simulink model "testwintrack2"  (R2021b)
settings: Solver=ode45  StartTime=0.0  StopTime=100  MaxStep=0.01  RelTol=1e-3
libraries: aerolibconvert2 x4, simulink x1
settings Model: Creator=cigla  LastModifiedBy=eforce

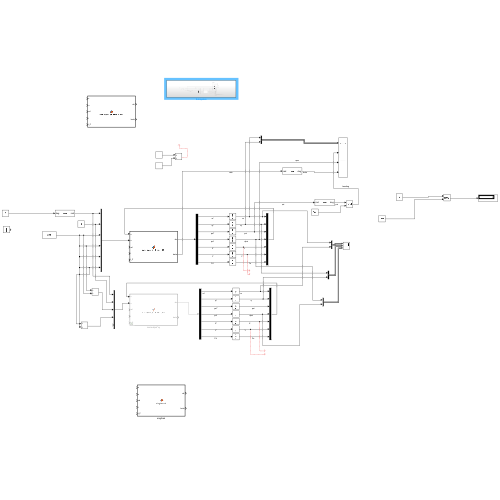
[thumbnail: Simulink's stored preview of the top-level diagram]
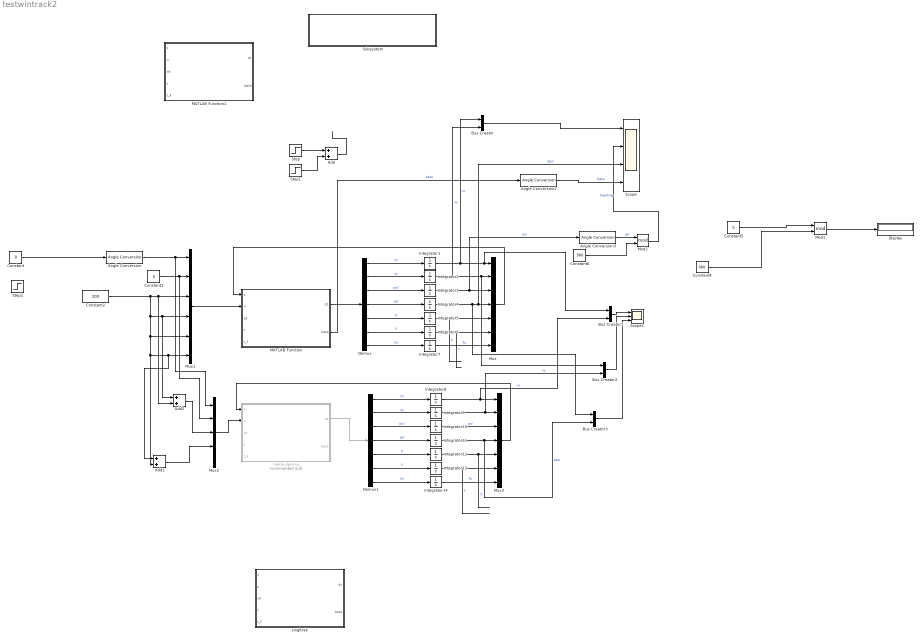
== system testwintrack2 ==
  Add : Sum
  Add1 : Sum
  Add2 : Sum
  Angle Conversion : aerolibconvert2/Angle Conversion  IU=deg  OU=rad
  Angle Conversion2 : aerolibconvert2/Angle Conversion  IU=rad  OU=deg
  Angle Conversion3 : aerolibconvert2/Angle Conversion  IU=rad  OU=deg
  Bus Creator{,1..3} (4 alike) : BusCreator  Inputs=2
  Constant : Constant  Value=0
  Constant1 : Constant  Value=0
  Constant2 : Constant  Value=200
  Constant4 : Constant  Value=360
  Constant5 : Constant  Value=5
  Constant6 : Constant  Value=360
  Demux : Demux  Outputs=7
  Demux1 : Demux  Outputs=7
  Display : Display
  Integrator{1..14} (14 alike) : Integrator
  MATLAB Function : MATLAB Function  TreatAsAtomicUnit=on
  MATLAB Function1 : MATLAB Function  TreatAsAtomicUnit=on
  Mod1 : Math  Operator=mod  SaturateOnIntegerOverflow=on
  Mod2 : Math  Operator=mod  SaturateOnIntegerOverflow=on
  Mux : Mux  Inputs=7
  Mux1 : Mux  Inputs=6
  Mux2 : Mux  Inputs=5
  Mux3 : Mux  Inputs=7
  Scope : Scope  NumInputPorts=4
  Scope1 : Scope  NumInputPorts=3
  Step : Step  Time=10  After=15  SampleTime=0
  Step1 : Step  Time=11  After=-30  SampleTime=0
  Step2 : Step  Time=10  After=20  SampleTime=0
  Subsystem : Subsystem
  nema dpsi*vy : MATLAB Function  Commented=on  TreatAsAtomicUnit=on
  singltrak : MATLAB Function  TreatAsAtomicUnit=on
  wires:
  MATLAB Function/1(dz) -> Demux/1
  Mux/1 -> MATLAB Function/1(z)
  Mux1/1 -> MATLAB Function/2(u)
  Demux/1 -> Integrator1/1  "vx'"
  Demux/2 -> Integrator2/1  "vy'"
  Demux/3 -> Integrator3/1  "psi''"
  Demux/4 -> Integrator4/1  "psi'"
  Demux/5 -> Integrator5/1  "X'"
  Demux/6 -> Integrator6/1  "Y'"
  Demux/7 -> Integrator7/1  "Fz'"
  Integrator1/1 -> Bus Creator/1, Bus Creator1/1, Mux/1  "vx"
  Integrator2/1 -> Bus Creator/2, Bus Creator2/1, Mux/2  "vy"
  Integrator7/1 -> Mux/7  "Fz"
  Integrator6/1 -> Mux/6  "Y"
  Integrator5/1 -> Mux/5  "X"
  Integrator4/1 -> Bus Creator3/1, Scope/3, Mux/4  "dpsi"
  Integrator3/1 -> Angle Conversion3/1, Mux/3  "psi"
  Add/1 -> ?
  Constant1/1 -> Mux2/2, Mux1/2
  Constant2/1 -> Add1/2, Add1/1, Mux1/6, Mux1/5, Add2/1, Mux1/4, Add2/2, Mux1/3
  Angle Conversion/1 -> Mux2/1, Mux1/1
  Step/1 -> Add/1
  Step1/1 -> Add/2
  Constant/1 -> Angle Conversion/1
  Bus Creator/1 -> Scope/1
  MATLAB Function/2(beta) -> Angle Conversion2/1  "beta"
  Angle Conversion2/1 -> Scope/4  "beta"
  Constant4/1 -> Mod1/2
  Constant5/1 -> Mod1/1
  Mod1/1 -> Display/1
  Angle Conversion3/1 -> Mod2/1  "psi"
  Constant6/1 -> Mod2/2
  Mod2/1 -> Scope/2  "heading"
  Add2/1 -> Mux2/3
  Add1/1 -> Mux2/4
  Mux2/1 -> nema dpsi*vy/2(u)
  Demux1/2 -> Integrator9/1  "vy'"
  Integrator14/1 -> Mux3/7  "Fz"
  Integrator12/1 -> Mux3/5  "X"
  Integrator10/1 -> Mux3/3  "psi"
  Integrator13/1 -> Mux3/6  "Y"
  Integrator9/1 -> Bus Creator2/2, Mux3/2  "vy"
  Demux1/5 -> Integrator12/1  "X'"
  Mux3/1 -> nema dpsi*vy/1(z)
  Demux1/7 -> Integrator14/1  "Fz'"
  Demux1/4 -> Integrator11/1  "psi'"
  Demux1/3 -> Integrator10/1  "psi''"
  Integrator11/1 -> Bus Creator3/2, Mux3/4  "dpsi"
  nema dpsi*vy/1(dz) -> Demux1/1
  Demux1/6 -> Integrator13/1  "Y'"
  Demux1/1 -> Integrator8/1  "vx'"
  Integrator8/1 -> Bus Creator1/2, Mux3/1  "vx"
  Bus Creator1/1 -> Scope1/1
  Bus Creator2/1 -> Scope1/2
  Bus Creator3/1 -> Scope1/3

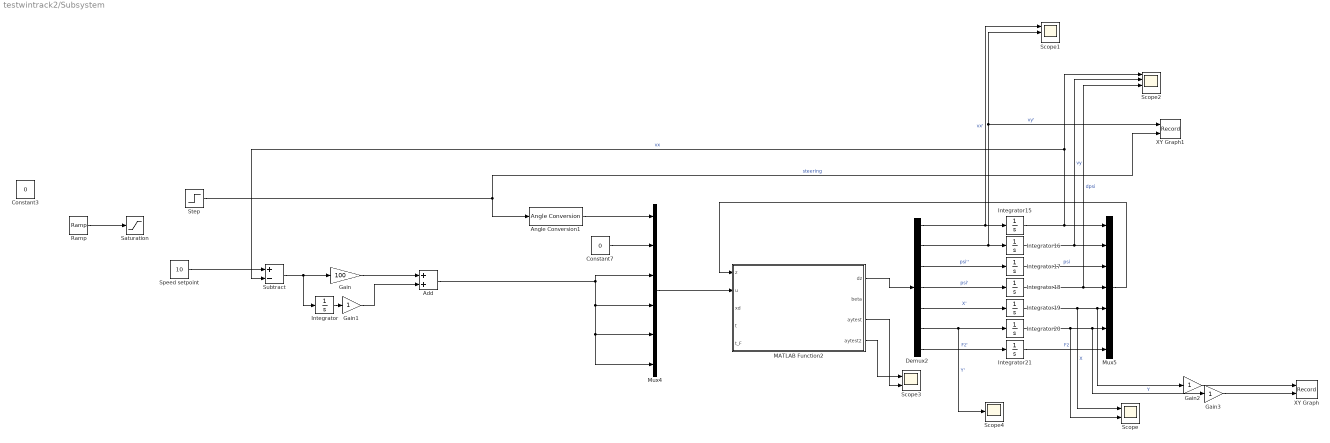
== system testwintrack2/Subsystem ==
  Add : Sum
  Angle Conversion1 : aerolibconvert2/Angle Conversion  IU=deg  OU=rad
  Constant3 : Constant  Value=0
  Constant7 : Constant  Value=0
  Demux2 : Demux  Outputs=7
  Gain : Gain  Gain=100
  Gain1 : Gain
  Gain2 : Gain
  Gain3 : Gain
  Integrator : Integrator  UpperSaturationLimit=10  LowerSaturationLimit=-10
  Integrator{15..21} (7 alike) : Integrator
  MATLAB Function2 : MATLAB Function  TreatAsAtomicUnit=on
  Mux4 : Mux  Inputs=6
  Mux5 : Mux  Inputs=7
  Ramp : simulink/Sources/Ramp  slope=1  start=30  InitialOutput=0
  Saturation : Saturate  UpperLimit=20  LowerLimit=-20
  Scope : Scope  NumInputPorts=2
  Scope1 : Scope  NumInputPorts=3
  Scope2 : Scope  NumInputPorts=4
  Scope3 : Scope  NumInputPorts=2
  Scope4 : Scope
  Speed setpoint : Constant  Value=10
  Step : Step  Time=10  After=10  SampleTime=0
  Subtract : Sum  Inputs=+-
  XY Graph : Record  FileSettingsInternal="{\"entries\":[{\"content\":{\"excelSettings\":{\"content\":{},\"type\":\"Streamout.ExcelSettings\"}},\"type\":\"Streamout.FileSettingStorage\",\"uuid\":\"7e0fd12c-69cb-45d7-9e50-e0eeec073e85\"}],\"packageUris\":[\"http://schema.mathworks.com/mf0/streamout_blocks/R2020a\"],\"version\":\"1.0\"}"  Layout=[1 1]  SignalsInternal="{\"entries\":[{\"content\":{\"signals\":[{\"content\":{\"blockPath\":[\"testwintrack2/Subsystem/XY Graph\"],\"channel\":[],\"dimensions\":[1],\"domain\":\"testwintrack2/Subsystem/XY Graph\",\"lineColor\":\"#a2142f\",\"plots\":[1],\"port\":1,\"sid\":[\"\"],\"signalID\":13090,\"signalName\":\"Gain2\"},\"type\":\"RecordBlkView.Signal\",\"uuid\":\"6ddc693e-96ce-4376-aff0-3416f7cc6428\"},{\"content\":{\"blockPath\":[\"testwintrack2/Subsystem/XY Graph\"],\"channel\":[],\"dimensions\":[1],\"domain\":\"testwintrack2/Subsystem/XY Graph\",\"lineColor\":\"#139fff\",\"plots\":[1],\"port\":2,\"sid\":[\"\"],\"signalID\":13094,\"signalName\":\"Gain3\"},\"type\":\"RecordBlkView.Signal\",\"uuid\":\"ac4ff5e3-5632-4bfd-aac4-21430a1220c0\"}]},\"type\":\"RecordBlkView.InputSignals\",\"uuid\":\"f93bda45-8b82-4e33-b9a7-b3c4e816161b\"}],\"packageUris\":[\"http://schema.mathworks.com/mf0/streamout_blocks/R2020a\"],\"version\":\"1.0\"}"  VisualizationBindings="{\"xyplotplugin\":{\"info\":[{\"series\":[{\"bindingParametersList\":[{\"parameter\":\"X-Axis\",\"signalID\":13094,\"signalName\":\"Gain3\"},{\"parameter\":\"Y-Axis\",\"signalID\":13090,\"signalName\":\"Gain2\"}],\"seriesID\":65193}],\"subplotID\":1}]}}"  CompatibilityTag=XY
  XY Graph1 : Record  FileSettingsInternal="{\"entries\":[{\"content\":{\"excelSettings\":{\"content\":{},\"type\":\"Streamout.ExcelSettings\"}},\"type\":\"Streamout.FileSettingStorage\",\"uuid\":\"7371816e-88d7-4fa3-a0a3-47bf26810cdb\"}],\"packageUris\":[\"http://schema.mathworks.com/mf0/streamout_blocks/R2020a\"],\"version\":\"1.0\"}"  Layout=[1 1]  SignalsInternal="{\"entries\":[{\"content\":{\"signals\":[{\"content\":{\"blockPath\":[\"testwintrack2/Subsystem/XY Graph1\"],\"channel\":[],\"dimensions\":[1],\"domain\":\"testwintrack2/Subsystem/XY Graph1\",\"lineColor\":\"#0072bd\",\"plots\":[1],\"port\":1,\"sid\":[\"\"],\"signalID\":13098,\"signalName\":\"vy'\"},\"type\":\"RecordBlkView.Signal\",\"uuid\":\"a0695c59-bb2a-41c0-904b-4f03a44cd8f8\"},{\"content\":{\"blockPath\":[\"testwintrack2/Subsystem/XY Graph1\"],\"channel\":[],\"dimensions\":[1],\"domain\":\"testwintrack2/Subsystem/XY Graph1\",\"lineColor\":\"#d95319\",\"plots\":[1],\"port\":2,\"sid\":[\"\"],\"signalID\":13102,\"signalName\":\"steering\"},\"type\":\"RecordBlkView.Signal\",\"uuid\":\"d041145a-05f3-4166-9c8f-163f23b06b29\"}]},\"type\":\"RecordBlkView.InputSignals\",\"uuid\":\"8f482f81-3f12-4fce-9d13-f56f0a380660\"}],\"packageUris\":[\"http://schema.mathworks.com/mf0/streamout_blocks/R2020a\"],\"version\":\"1.0\"}"  VisualizationBindings="{\"xyplotplugin\":{\"info\":[{\"series\":[{\"bindingParametersList\":[{\"parameter\":\"X-Axis\",\"signalID\":13098,\"signalName\":\"vy'\"},{\"parameter\":\"Y-Axis\",\"signalID\":13102,\"signalName\":\"steering\"}],\"seriesID\":246}],\"subplotID\":1}]}}"  CompatibilityTag=XY
  wires:
  Integrator15/1 -> Subtract/2, Scope2/1, Mux5/1  "vx"
  Integrator18/1 -> Scope2/3, Mux5/4  "dpsi"
  Integrator20/1 -> Scope/2, Gain3/1, Mux5/6  "Y"
  Demux2/1 -> Scope1/1, Integrator15/1  "vx'"
  Integrator16/1 -> Scope2/2, Mux5/2  "vy"
  Ramp/1 -> Saturation/1
  Demux2/3 -> Integrator17/1  "psi''"
  Integrator17/1 -> Mux5/3  "psi"
  Integrator19/1 -> Scope/1, Gain2/1, Mux5/5  "X"
  Integrator21/1 -> Mux5/7  "Fz"
  Mux4/1 -> MATLAB Function2/2(u)
  Mux5/1 -> MATLAB Function2/1(z)
  Add/1 -> Mux4/6, Mux4/5, Mux4/4, Mux4/3
  Constant7/1 -> Mux4/2
  Demux2/2 -> XY Graph1/1, Scope1/2, Integrator16/1  "vy'"
  Demux2/6 -> Scope4/1, Integrator20/1  "Y'"
  Angle Conversion1/1 -> Mux4/1
  MATLAB Function2/1(dz) -> Demux2/1
  Demux2/7 -> Integrator21/1  "Fz'"
  Demux2/5 -> Integrator19/1  "X'"
  Demux2/4 -> Integrator18/1  "psi'"
  Speed setpoint/1 -> Subtract/1
  Subtract/1 -> Integrator/1, Gain/1
  Gain/1 -> Add/1
  Gain1/1 -> Add/2
  Integrator/1 -> Gain1/1
  Step/1 -> Angle Conversion1/1, XY Graph1/2  "steering"
  Gain2/1 -> XY Graph/1
  Gain3/1 -> XY Graph/2
  MATLAB Function2/3(aytest) -> Scope3/2
  MATLAB Function2/4(aytest2) -> Scope3/1

== matlab function testwintrack2/singltrak ==
  data: z input size=7; u input size=6; dz output size=7; xd input; t input; t_F input; beta output
function [dz, beta]= singletrack(z, u, xd, t, t_F)
% z = [vx; vy; psi; dpsidt; X; Y], vx-longitudinal velocity, vy-lateral velocity, psi-angular position of the car with respect to the inertial frame, X and Y are coordinates of the car in the inertial frame
% u = [delta_f; delta_r; Ff; Fr], delta_f - steering angle of the front wheel, delta_r - steering angle of the rear wheel (NOT IMPLEMENTED YET), Ff - force acting on the front wheel in the longitudinal direction, Fr - force acting on the rear wheel in the longitudinal direction
% car - structure containing parameters of the car model




%%%%%%%%%%%%%%%%%%%% Car parameters %%%%%%%%%%%%%%%%%%%%
m            = 280;                      % weight of the car [kg]
Izz          = 100;                      % moment of inertia [kg m^2]
wheelbase    = 1.525;                    % distance between the front and rear axles [m];
track        = 0;                      % distance between right and left wheel
distribution = 50;                       % COG distribution percent on rear
COG          = wheelbase*(distribution/100);     % distance of Center Of Gravity (COG) from the front axle [m];
l_f          = COG;                  % distance of the front axle form the COG [m];
l_r          = wheelbase - COG;  % distance of the rear axle form the COG [m];
COGz         = 0.3;                      % height of COG from ground
wheelradius  = 0.205;                    % radius of the wheels [m]
steeringAngle_max = 20/180*pi;           % Maximum allowed steering angle
steeringAngle_maxRate = 200/180*pi;      % Maximum allowed steering angle [rad/s]
%% Motor parameters
Mf_max       = 29.1 * 2 * 11.46;         % maximum torque generated by a motor on the front axle [Nm]
Mf_slewRate  = 100;                      % maximum slew rate of the generated torque on the rear axle [Nm/s]
Mr_max       = 29.1 * 2 * 11.46;         % maximum torque generated by a motor on the rear axle [Nm]
Mr_slewRate  = 100;                      % maximum slew rate of the generated torque on the rear axle [Nm/s]
Yt_max       = (Mf_max/wheelradius + Mr_max/wheelradius)*track;                    % maximum Yaw moment
PwrMax       = 80000;
PwrMin       = -40000;
maxSpeed     = 40;                        %m/s


%% Tire and suspension parameters
E = 0.23;
D = 1;
B = 0.3;
C = 1;




Sus_t = 100;                          % suspension time constant for 1st order system
tire_fxFactor = 1.5 ;                 % max Fx = Fz * tire_fxFactor
tire_fyFactor = 1.3 ;                 % max Fy = Fz * tire_fyFactor
%ftire = @(alph, Fz, p)(alph/pi*180)* Fz * tire_stifness ; % 
%ftire = @(alph,Fz, p)  Fz* D*sin(C*atan(B*(alph/pi*180)  - E*atan(B*(alph/pi*180))));
ftire = @(alph, Fz)(alph/pi.*180)./15.* Fz .* tire_fyFactor ; % 

%% Aerodynamics parameters
CL  = -4.15;
CD  = 1.55;
A   = 1;
COP = 0.5;    % Center of pressure on rear ratio

%% environment parameters
g = 9.81;
airDensity = 1.225;






    Ft = u;

delta_f = Ft(1);
delta_r = Ft(2);
Ff      = Ft(3);
Fr      = Ft(4);
Yt      = Ft(5);

% Extract the states from z
v_x  = z(1);
v_y  = z(2);
psi  = z(3);
dpsi = z(4);
X    = z(5);
Y    = z(6);
Fz   = z(7);

% Compute the slip angles
% alpha_f_old = delta_f - atan2(v_y + l_f*dpsi, v_x);
alpha_f = -atan2((v_y + l_f*dpsi)*cos(delta_f) - v_x*sin(delta_f) ,...
                 (v_y + l_f*dpsi)*sin(delta_f) + v_x*cos(delta_f));
% alpha_r_old = delta_r - atan2(v_y - l_r*dpsi, v_x);
alpha_r = -atan2((v_y - l_r*dpsi)*cos(delta_r) - v_x*sin(delta_r) ,...
                 (v_y - l_r*dpsi)*sin(delta_r) + v_x*cos(delta_r));
% [alpha_f_old, alpha_f, alpha_f_old - alpha_f, alpha_r_old, alpha_r, alpha_r_old - alpha_r]
% Compute the forces acting on the wheels

Fz_aero = 0.5*airDensity*CL*A*v_x.^2;

Fz_f = m/2 * g ;%- Fz - Fz_aero * (1-COP);
Fz_r = m/2 * g ;%+ Fz - Fz_aero * COP;

F_fy = ftire(alpha_f,Fz_f);
F_ry = ftire(alpha_r,Fz_r);
F_fx = Ff;
F_rx = Fr;

% Compute quantities need for the change of the position in the inertial frame
v = sqrt(v_x^2 + v_y^2);
beta = atan2(v_y, v_x);

dvx = 1/m  * (F_rx*cos(delta_r) - F_ry*sin(delta_r) + F_fx*cos(delta_f) - F_fy*sin(delta_f) - 0.0*airDensity*CD*A*v_x^2) + dpsi*v_y;
dz = [... 
dvx;                                                                                                                          % v_x/dt
1/m  * (F_rx*sin(delta_r) + F_ry*cos(delta_r) + F_fx*sin(delta_f) + F_fy*cos(delta_f)) - dpsi*v_x;                        % v_y/dt  
dpsi;                                                                                                                         % psi/dt
1/Izz * (l_f*F_fx*sin(delta_f) + l_f*F_fy*cos(delta_f) - l_r*F_rx*sin(delta_r) - l_r*F_ry*cos(delta_r)) %+ Yt/Izz;  % dpsi
v*cos(psi + beta);                                                                                                            % X/dt
v*sin(psi + beta);                                                                                                            % Y/dt
(dvx*COGz/wheelbase*m-Fz)/Sus_t;                                                                              %Fz/dt  
];

end

== matlab function testwintrack2/MATLAB Function ==
  data: z input size=7; u input size=6; dz output size=7; xd input; t input; t_F input; beta output
function [dz, beta]= twinRaceCar_time_ODE(z, u, xd, t, t_F)
% z = [vx; vy; psi; dpsidt; X; Y], vx-longitudinal velocity, vy-lateral velocity, psi-angular position of the car with respect to the inertial frame, X and Y are coordinates of the car in the inertial frame
% u = [delta_f; delta_r; Ff; Fr], delta_f - steering angle of the front wheel, delta_r - steering angle of the rear wheel (NOT IMPLEMENTED YET), Ff - force acting on the front wheel in the longitudinal direction, Fr - force acting on the rear wheel in the longitudinal direction
% car - structure containing parameters of the car model




%%%%%%%%%%%%%%%%%%%% Car parameters %%%%%%%%%%%%%%%%%%%%
tracks       = 2;
m            = 280;                      % weight of the car [kg]
Izz          = 100;                      % moment of inertia [kg m^2]
wheelbase    = 1.525;                    % distance between the front and rear axles [m];
track        = 1.2;                      % distance between right and left wheel
COGr         = 0.5;                       % COG distribution 0-1 scale on rear
COG          = wheelbase*(COGr); % distance of Center Of Gravity (COG) from the front axle [m];
l_f          = COG;                  % distance of the front axle form the COG [m];
l_r          = wheelbase - COG;  % distance of the rear axle form the COG [m];
COGz         = 0.3;                      % height of COG from ground
wheelradius  = 0.205;                    % radius of the wheels [m]
steeringAngle_max = 20/180*pi;           % Maximum allowed steering angle
steeringAngle_maxRate = 400/180*pi;      % Maximum allowed steering angle [rad/s]
%% Motor parameters
Mf_max       = 29.1 * 2/tracks * 11.46;         % maximum torque generated by a motor on the front axle [Nm]
Mf_slewRate  = 16000;                      % maximum slew rate of the generated torque on the rear axle [Nm/s]0.5 je ca 1000/s idk preco
Mf_jerk       = 800;                           % 1000 bolo cca okay
Mr_max       = 29.1 * 2/tracks * 11.46;         % maximum torque generated by a motor on the rear axle [Nm]
Mr_slewRate  = 100;                      % maximum slew rate of the generated torque on the rear axle [Nm/s]
Yt_max       = (Mf_max/wheelradius + Mr_max/wheelradius)*track;                    % maximum Yaw moment
PwrMax       = 80000;
PwrMin       = -40000;
maxSpeed     = 40;                        %m/sftire


%% Tire and suspension parameters
E = 0.23;
D = 1;
B = 0.3;
C = 1;


Sus_t = 0.3;                          % suspension time constant for 1st order system
tire_fxFactor = 1.5 ;                 % max Fx = Fz * tire_fxFactor
tire_fyFactor = 1.3 ;                 % max Fy = Fz * tire_fyFactor
%ftire = @(alph, Fz, p)(alph/pi*180)* Fz * tire_stifness ; %
%ftire = @(alph,Fz, p)  Fz* D*sin(C*atan(B*(alph/pi*180)  - E*atan(B*(alph/pi*180))));
ftire = @(alph, Fz)(alph./pi.*180)./15.* Fz .* tire_fyFactor ; %

%% Aerodynamics parameters
CL  = -4.15;
CD  = 1.55;
A   = 1;
COP = 0.5;    % Center of pressure on rear ratio
wingLength_f = 0.9;

%% environment parameters
g = 9.81;
airDensity = 1.225;


    Ft = u;

% Extract the controls from F
delta_f  = Ft(1);
delta_r  = Ft(2);
Fx_fl     = Ft(3);
Fx_fr     = Ft(4);
Fx_rl     = Ft(5);
Fx_rr     = Ft(6);


%% Extract the states from z
v_x  = z(1);
v_y  = z(2);
psi  = z(3);
dpsi = z(4);
X    = z(5);
Y    = z(6);
Fz   = z(7);

%% Compute the slip angles
%% Compute the slip angles
%% initialize matrices, origin of car is in COG
v = [v_x v_y 0];
dpsiv = [ 0 0 dpsi];
pos_fr = [  l_f  -track/2 0];
pos_fl = [  l_f   track/2 0];
pos_rr = [ -l_r -track/2 0];
pos_rl = [ -l_r  track/2 0];

%% Calculate vectors at uprights
velocityUpright_fl = v + cross(dpsiv,pos_fl);
velocityUpright_fr = v + cross(dpsiv,pos_fr);
velocityUpright_rl = v + cross(dpsiv,pos_rl);
velocityUpright_rr = v + cross(dpsiv,pos_rr);

%% Define Rotation matrices
rotate_f = [
    cos(delta_f) -sin(delta_f) 0
    sin(delta_f) cos(delta_f)  0
    0            0             0
    ];
rotate_r = [
    cos(delta_r) -sin(delta_r) 0
    sin(delta_r) cos(delta_r)  0
    0            0             0
    ];

%% Calculate wheel velocity in wheel frames
velocityWheel_fl = velocityUpright_fl * rotate_f;
velocityWheel_fr = velocityUpright_fr * rotate_f;
velocityWheel_rl = velocityUpright_rl * rotate_r;
velocityWheel_rr = velocityUpright_rr * rotate_r;


%% Calculate alphas
alpha_fl = -atan2(velocityWheel_fl(2),velocityWheel_fl(1));
alpha_fr = -atan2(velocityWheel_fr(2),velocityWheel_fr(1));
alpha_rl = -atan2(velocityWheel_rl(2),velocityWheel_rl(1));
alpha_rr = -atan2(velocityWheel_rr(2),velocityWheel_rr(1));


%% Compute the forces acting on the wheels
Fz_aero = 0.5*airDensity*CL*A*v_x.^2;
Fz_f = m/2*(1-COGr) * g - Fz/2 - Fz_aero/2 * (1-COP);
Fz_r = m/2*(COGr)   * g + Fz/2 - Fz_aero/2 * COP;

Fy_fl = ftire(alpha_fl,Fz_f);
Fy_fr = ftire(alpha_fr,Fz_f);
Fy_rl = ftire(alpha_rl,Fz_r);
Fy_rr = ftire(alpha_rr,Fz_r);

%% Projection of forces from steered wheels to uprights
projection_f = [
    cos(delta_f)      sin(delta_f)
    -sin(delta_f)     cos(delta_f)   
    ];
projection_r = [
    cos(delta_r)      sin(delta_r)
    -sin(delta_r)     cos(delta_r)   
    ];
%% Forces acting on uprights
F_fl = [Fx_fl Fy_fl] * projection_f;
F_fr = [Fx_fr Fy_fr] * projection_f;
F_rl = [Fx_rl Fy_rl] * projection_r;
F_rr = [Fx_rr Fy_rr] * projection_r;

F_drag = 0.5*airDensity*CD*A*v_x^2;
% Compute quantities need for the change of the position in the inertial frame
v = sqrt(v_x^2 + v_y^2);
beta = atan2(v_y, v_x);

M = (F_fr(1) + F_rr(1) - F_fl(1) - F_rl(1))*track/2 +... % Forward forces create Moment
    (F_fr(2) + F_fl(2)) * l_f...                         % Lateral forces from front tires
   -(F_rr(2) + F_rl(2)) * l_r;                          % Lateral forces from rear tires

Fx = F_fr(1) + F_rr(1) + F_fl(1) + F_rl(1)- F_drag;         % Longitudinal force from wheels and drag
Fy = F_fr(2) + F_rr(2) + F_fl(2) + F_rl(2);                  % Lateral force


%dvx = 1/m  * (F_rx*cos(delta_r) - F_ry*sin(delta_r) + F_fx*cos(delta_f) - F_fy*sin(delta_f) - 0.5*airDensity*CD*A*v_x^2) + dpsi*v_y;
dz = [... 
Fx/m  + dpsi*v_y                                                                                                                      % v_x/dt
Fy/m  - dpsi*v_x                      % v_y/dt  
dpsi;                                                                                                                         % psi/dt
M/Izz   % dpsi
v*cos(psi + beta);                                                                                                            % X/dt
v*sin(psi + beta);                                                                                                            % Y/dt
((Fx/m + dpsi*v_y) *COGz/wheelbase*m-Fz)/Sus_t;                                                                              %Fz/dt  
];
end

== matlab function testwintrack2/nema dpsi*vy ==
  data: z input size=7; u input size=6; dz output size=7; xd input; t input; t_F input; beta output
function [dz, beta]= twinRaceCar_time_ODE(z, u, xd, t, t_F)
% z = [vx; vy; psi; dpsidt; X; Y], vx-longitudinal velocity, vy-lateral velocity, psi-angular position of the car with respect to the inertial frame, X and Y are coordinates of the car in the inertial frame
% u = [delta_f; delta_r; Ff; Fr], delta_f - steering angle of the front wheel, delta_r - steering angle of the rear wheel (NOT IMPLEMENTED YET), Ff - force acting on the front wheel in the longitudinal direction, Fr - force acting on the rear wheel in the longitudinal direction
% car - structure containing parameters of the car model




%%%%%%%%%%%%%%%%%%%% Car parameters %%%%%%%%%%%%%%%%%%%%
m            = 280;                      % weight of the car [kg]
Izz          = 100;                      % moment of inertia [kg m^2]
wheelbase    = 1.525;                    % distance between the front and rear axles [m];
track        = 0;                      % distance between right and left wheel
distribution = 50;                       % COG distribution percent on rear
COG          = wheelbase*(distribution/100);     % distance of Center Of Gravity (COG) from the front axle [m];
l_f          = COG;                  % distance of the front axle form the COG [m];
l_r          = wheelbase - COG;  % distance of the rear axle form the COG [m];
COGz         = 0.3;                      % height of COG from ground
wheelradius  = 0.205;                    % radius of the wheels [m]
steeringAngle_max = 20/180*pi;           % Maximum allowed steering angle
steeringAngle_maxRate = 200/180*pi;      % Maximum allowed steering angle [rad/s]
%% Motor parameters
Mf_max       = 29.1 * 2 * 11.46;         % maximum torque generated by a motor on the front axle [Nm]
Mf_slewRate  = 100;                      % maximum slew rate of the generated torque on the rear axle [Nm/s]
Mr_max       = 29.1 * 2 * 11.46;         % maximum torque generated by a motor on the rear axle [Nm]
Mr_slewRate  = 100;                      % maximum slew rate of the generated torque on the rear axle [Nm/s]
Yt_max       = (Mf_max/wheelradius + Mr_max/wheelradius)*track;                    % maximum Yaw moment
PwrMax       = 80000;
PwrMin       = -40000;
maxSpeed     = 40;                        %m/s


%% Tire and suspension parameters
E = 0.23;
D = 1;
B = 0.3;
C = 1;




Sus_t = 100;                          % suspension time constant for 1st order system
tire_fxFactor = 1.5 ;                 % max Fx = Fz * tire_fxFactor
tire_fyFactor = 1.3 ;                 % max Fy = Fz * tire_fyFactor
%ftire = @(alph, Fz, p)(alph/pi*180)* Fz * tire_stifness ; % 
%ftire = @(alph,Fz, p)  Fz* D*sin(C*atan(B*(alph/pi*180)  - E*atan(B*(alph/pi*180))));
ftire = @(alph, Fz)(alph/pi.*180)./15.* Fz .* tire_fyFactor ; % 

%% Aerodynamics parameters
CL  = -4.15;
CD  = 1.55;
A   = 1;
COP = 0.5;    % Center of pressure on rear ratio

%% environment parameters
g = 9.81;
airDensity = 1.225;






    Ft = u;

% Extract the controls from F
delta_f = Ft(1);
delta_r = Ft(2);
Ff_l     = Ft(3);
Ff_r     = Ft(4);
Fr_l     = Ft(5);
Fr_r     = Ft(6);


%% Extract the states from z
v_x  = z(1);
v_y  = z(2);
psi  = z(3);
dpsi = z(4);
X    = z(5);
Y    = z(6);
Fz   = z(7);

%% Compute the slip angles
%% Compute the slip angles
%% initialize matrices, origin of car is in COG
v = [v_x v_y 0];
dpsiv = [ 0 0 dpsi];
pos_fr = [  l_f  -track/2 0];
pos_fl = [  l_f   track/2 0];
pos_rr = [ -l_r -track/2 0];
pos_rl = [ -l_r  track/2 0];

%% Calculate vectors at uprights
velocityUpright_fl = v + cross(dpsiv,pos_fl);
velocityUpright_fr = v + cross(dpsiv,pos_fr);
velocityUpright_rl = v + cross(dpsiv,pos_rl);
velocityUpright_rr = v + cross(dpsiv,pos_rr);

%% Define Rotation matrices
rotate_f = [
    cos(delta_f) -sin(delta_f) 0
    sin(delta_f) cos(delta_f)  0
    0            0             0
    ];
rotate_r = [
    cos(delta_r) -sin(delta_r) 0
    sin(delta_r) cos(delta_r)  0
    0            0             0
    ];

%% Calculate wheel velocity in wheel frames
velocityWheel_fl = velocityUpright_fl * rotate_f;
velocityWheel_fr = velocityUpright_fr * rotate_f;
velocityWheel_rl = velocityUpright_rl * rotate_r;
velocityWheel_rr = velocityUpright_rr * rotate_r;


%% Calculate alphas
alpha_fl = -atan2(velocityWheel_fl(2),velocityWheel_fl(1));
alpha_fr = -atan2(velocityWheel_fr(2),velocityWheel_fr(1));
alpha_rl = -atan2(velocityWheel_rl(2),velocityWheel_rl(1));
alpha_rr = -atan2(velocityWheel_rr(2),velocityWheel_rr(1));


%% Compute the forces acting on the wheels
Fz_aero = 0.5*airDensity*CL*A*v_x.^2;
Fz_f = m/4 * g;% - Fz/2 - Fz_aero/2 * (1-COP);
Fz_r = m/4 * g; %+ Fz/2 - Fz_aero/2 * COP;

Fy_fl = ftire(alpha_fl,Fz_f);
Fy_fr = ftire(alpha_fr,Fz_f);
Fy_rl = ftire(alpha_rl,Fz_r);
Fy_rr = ftire(alpha_rr,Fz_r);

Fx_fl = Ff_l;
Fx_fr = Ff_r;
Fx_rl = Fr_l;
Fx_rr = Fr_r;
%% Projection of forces from steered wheels to uprights
projection_f = [
    cos(delta_f)      sin(delta_f)
    -sin(delta_f)     cos(delta_f)   
    ];
projection_r = [
    cos(delta_r)      sin(delta_r)
    -sin(delta_r)     cos(delta_r)   
    ];
%% Forces acting on uprights
F_fl = [Fx_fl Fy_fl] * projection_f;
F_fr = [Fx_fr Fy_fr] * projection_f;
F_rl = [Fx_rl Fy_rl] * projection_r;
F_rr = [Fx_rr Fy_rr] * projection_r;

F_drag = 0.0*airDensity*CD*A*v_x^2;
% Compute quantities need for the change of the position in the inertial frame
v = sqrt(v_x^2 + v_y^2);
beta = atan2(v_y, v_x);

M = (F_fr(1) + F_rr(1) - F_fl(1) - F_rl(1))*track/2*0 +... % Forward forces create Moment
    (F_fr(2) + F_fl(2)) * l_f...                         % Lateral forces from front tires
   -(F_rr(2) + F_rl(2)) * l_r;                          % Lateral forces from rear tires

Fx = F_fr(1) + F_rr(1) + F_fl(1) + F_rl(1)- F_drag;         % Longitudinal force from wheels and drag
Fy = F_fr(2) + F_rr(2) + F_fl(2) + F_rl(2);                  % Lateral force


%dvx = 1/m  * (F_rx*cos(delta_r) - F_ry*sin(delta_r) + F_fx*cos(delta_f) - F_fy*sin(delta_f) - 0.5*airDensity*CD*A*v_x^2) + dpsi*v_y;
dz = [... 
Fx/m                                                                                                                     % v_x/dt
Fy/m  - dpsi*v_x                      % v_y/dt  
dpsi;                                                                                                                         % psi/dt
M/Izz   % dpsi
v*cos(psi + beta);                                                                                                            % X/dt
v*sin(psi + beta);                                                                                                            % Y/dt
((Fx/m + dpsi*v_y) *COGz/wheelbase*m-Fz)/Sus_t;                                                                              %Fz/dt  
];
end

== matlab function testwintrack2/MATLAB Function1 ==
  data: z input size=7; u input size=6; dz output size=7; xd input; t input; t_F input; beta output
function [dz, beta]= twinRaceCar_time_ODE(z, u, xd, t, t_F)
% z = [vx; vy; psi; dpsidt; X; Y], vx-longitudinal velocity, vy-lateral velocity, psi-angular position of the car with respect to the inertial frame, X and Y are coordinates of the car in the inertial frame
% u = [delta_f; delta_r; Ff; Fr], delta_f - steering angle of the front wheel, delta_r - steering angle of the rear wheel (NOT IMPLEMENTED YET), Ff - force acting on the front wheel in the longitudinal direction, Fr - force acting on the rear wheel in the longitudinal direction
% car - structure containing parameters of the car model




%%%%%%%%%%%%%%%%%%%% Car parameters %%%%%%%%%%%%%%%%%%%%
tracks       = 2;
m            = 280;                      % weight of the car [kg]
Izz          = 100;                      % moment of inertia [kg m^2]
wheelbase    = 1.525;                    % distance between the front and rear axles [m];
track        = 1.2;                      % distance between right and left wheel
COGr         = 0.5;                       % COG distribution 0-1 scale on rear
COG          = wheelbase*(COGr); % distance of Center Of Gravity (COG) from the front axle [m];
l_f          = COG;                  % distance of the front axle form the COG [m];
l_r          = wheelbase - COG;  % distance of the rear axle form the COG [m];
COGz         = 0.3;                      % height of COG from ground
wheelradius  = 0.205;                    % radius of the wheels [m]
steeringAngle_max = 20/180*pi;           % Maximum allowed steering angle
steeringAngle_maxRate = 400/180*pi;      % Maximum allowed steering angle [rad/s]
%% Motor parameters
Mf_max       = 29.1 * 2/tracks * 11.46;         % maximum torque generated by a motor on the front axle [Nm]
Mf_slewRate  = 16000;                      % maximum slew rate of the generated torque on the rear axle [Nm/s]0.5 je ca 1000/s idk preco
Mf_jerk       = 800;                           % 1000 bolo cca okay
Mr_max       = 29.1 * 2/tracks * 11.46;         % maximum torque generated by a motor on the rear axle [Nm]
Mr_slewRate  = 100;                      % maximum slew rate of the generated torque on the rear axle [Nm/s]
Yt_max       = (Mf_max/wheelradius + Mr_max/wheelradius)*track;                    % maximum Yaw moment
PwrMax       = 80000;
PwrMin       = -40000;
maxSpeed     = 40;                        %m/sftire


%% Tire and suspension parameters
E = 0.23;
D = 1;
B = 0.3;
C = 1;


Sus_t = 0.3;                          % suspension time constant for 1st order system
tire_fxFactor = 1.5 ;                 % max Fx = Fz * tire_fxFactor
tire_fyFactor = 1.3 ;                 % max Fy = Fz * tire_fyFactor
%ftire = @(alph, Fz, p)(alph/pi*180)* Fz * tire_stifness ; %
%ftire = @(alph,Fz, p)  Fz* D*sin(C*atan(B*(alph/pi*180)  - E*atan(B*(alph/pi*180))));
ftire = @(alph, Fz)(alph./pi.*180)./15.* Fz .* tire_fyFactor ; %

%% Aerodynamics parameters
CL  = -4.15;
CD  = 1.55;
A   = 1;
COP = 0.5;    % Center of pressure on rear ratio
wingLength_f = 0.9;

%% environment parameters
g = 9.81;
airDensity = 1.225;


    Ft = u;

% Extract the controls from F
delta_f  = Ft(1);
delta_r  = Ft(2);
Fx_fl     = Ft(3);
Fx_fr     = Ft(4);
Fx_rl     = Ft(5);
Fx_rr     = Ft(6);


%% Extract the states from z
v_x  = z(1);
v_y  = z(2);
psi  = z(3);
dpsi = z(4);
X    = z(5);
Y    = z(6);
Fz   = z(7);

%% Compute the slip angles
%% Compute the slip angles
%% initialize matrices, origin of car is in COG
v = [v_x v_y 0];
dpsiv = [ 0 0 dpsi];
pos_fr = [  l_f  -track/2 0];
pos_fl = [  l_f   track/2 0];
pos_rr = [ -l_r -track/2 0];
pos_rl = [ -l_r  track/2 0];

%% Calculate vectors at uprights
velocityUpright_fl = v + cross(dpsiv,pos_fl);
velocityUpright_fr = v + cross(dpsiv,pos_fr);
velocityUpright_rl = v + cross(dpsiv,pos_rl);
velocityUpright_rr = v + cross(dpsiv,pos_rr);

%% Define Rotation matrices
rotate_f = [
    cos(delta_f) -sin(delta_f) 0
    sin(delta_f) cos(delta_f)  0
    0            0             0
    ];
rotate_r = [
    cos(delta_r) -sin(delta_r) 0
    sin(delta_r) cos(delta_r)  0
    0            0             0
    ];

%% Calculate wheel velocity in wheel frames
velocityWheel_fl = velocityUpright_fl * rotate_f;
velocityWheel_fr = velocityUpright_fr * rotate_f;
velocityWheel_rl = velocityUpright_rl * rotate_r;
velocityWheel_rr = velocityUpright_rr * rotate_r;


%% Calculate alphas
alpha_fl = -atan2(velocityWheel_fl(2),velocityWheel_fl(1));
alpha_fr = -atan2(velocityWheel_fr(2),velocityWheel_fr(1));
alpha_rl = -atan2(velocityWheel_rl(2),velocityWheel_rl(1));
alpha_rr = -atan2(velocityWheel_rr(2),velocityWheel_rr(1));


%% Compute the forces acting on the wheels
Fz_aero = 0.5*airDensity*CL*A*v_x.^2;
Fz_f = m/2*(1-COGr) * g - Fz/2 - Fz_aero/2 * (1-COP);
Fz_r = m/2*(COGr)   * g + Fz/2 - Fz_aero/2 * COP;

Fy_fl = ftire(alpha_fl,Fz_f);
Fy_fr = ftire(alpha_fr,Fz_f);
Fy_rl = ftire(alpha_rl,Fz_r);
Fy_rr = ftire(alpha_rr,Fz_r);

%% Projection of forces from steered wheels to uprights
projection_f = [
    cos(delta_f)      sin(delta_f)
    -sin(delta_f)     cos(delta_f)   
    ];
projection_r = [
    cos(delta_r)      sin(delta_r)
    -sin(delta_r)     cos(delta_r)   
    ];
%% Forces acting on uprights
F_fl = [Fx_fl Fy_fl] * projection_f;
F_fr = [Fx_fr Fy_fr] * projection_f;
F_rl = [Fx_rl Fy_rl] * projection_r;
F_rr = [Fx_rr Fy_rr] * projection_r;

F_drag = 0.5*airDensity*CD*A*v_x^2;
% Compute quantities need for the change of the position in the inertial frame
v = sqrt(v_x^2 + v_y^2);
beta = atan2(v_y, v_x);

M = (F_fr(1) + F_rr(1) - F_fl(1) - F_rl(1))*track/2 +... % Forward forces create Moment
    (F_fr(2) + F_fl(2)) * l_f...                         % Lateral forces from front tires
   -(F_rr(2) + F_rl(2)) * l_r;                          % Lateral forces from rear tires

Fx = F_fr(1) + F_rr(1) + F_fl(1) + F_rl(1)- F_drag;         % Longitudinal force from wheels and drag
Fy = F_fr(2) + F_rr(2) + F_fl(2) + F_rl(2);                  % Lateral force


%dvx = 1/m  * (F_rx*cos(delta_r) - F_ry*sin(delta_r) + F_fx*cos(delta_f) - F_fy*sin(delta_f) - 0.5*airDensity*CD*A*v_x^2) + dpsi*v_y;
dz = [... 
Fx/m  + dpsi*v_y                                                                                                                      % v_x/dt
Fy/m  - dpsi*v_x                      % v_y/dt  
dpsi;                                                                                                                         % psi/dt
M/Izz   % dpsi
v*cos(psi + beta);                                                                                                            % X/dt
v*sin(psi + beta);                                                                                                            % Y/dt
((Fx/m + dpsi*v_y) *COGz/wheelbase*m-Fz)/Sus_t;                                                                              %Fz/dt  
];
end

== matlab function testwintrack2/Subsystem/MATLAB Function2 ==
  data: z input size=7; u input size=6; dz output size=7; xd input; t input; t_F input; beta output; aytest output; aytest2 output
function [dz, beta, aytest, aytest2]= twinRaceCar_time_ODE(z, u, xd, t, t_F)
% z = [vx; vy; psi; dpsidt; X; Y], vx-longitudinal velocity, vy-lateral velocity, psi-angular position of the car with respect to the inertial frame, X and Y are coordinates of the car in the inertial frame
% u = [delta_f; delta_r; Ff; Fr], delta_f - steering angle of the front wheel, delta_r - steering angle of the rear wheel (NOT IMPLEMENTED YET), Ff - force acting on the front wheel in the longitudinal direction, Fr - force acting on the rear wheel in the longitudinal direction
% car - structure containing parameters of the car model




%%%%%%%%%%%%%%%%%%%% Car parameters %%%%%%%%%%%%%%%%%%%%
tracks       = 2;
m            = 280;                      % weight of the car [kg]
Izz          = 100;                      % moment of inertia [kg m^2]
wheelbase    = 1.525;                    % distance between the front and rear axles [m];
track        = 1.2;                      % distance between right and left wheel
COGr         = 0.5;                       % COG distribution 0-1 scale on rear
COG          = wheelbase*(COGr); % distance of Center Of Gravity (COG) from the front axle [m];
l_f          = COG;                  % distance of the front axle form the COG [m];
l_r          = wheelbase - COG;  % distance of the rear axle form the COG [m];
COGz         = 0.3;                      % height of COG from ground
wheelradius  = 0.205;                    % radius of the wheels [m]
steeringAngle_max = 20/180*pi;           % Maximum allowed steering angle
steeringAngle_maxRate = 400/180*pi;      % Maximum allowed steering angle [rad/s]
%% Motor parameters
Mf_max       = 29.1 * 2/tracks * 11.46;         % maximum torque generated by a motor on the front axle [Nm]
Mf_slewRate  = 16000;                      % maximum slew rate of the generated torque on the rear axle [Nm/s]0.5 je ca 1000/s idk preco
Mf_jerk       = 800;                           % 1000 bolo cca okay
Mr_max       = 29.1 * 2/tracks * 11.46;         % maximum torque generated by a motor on the rear axle [Nm]
Mr_slewRate  = 100;                      % maximum slew rate of the generated torque on the rear axle [Nm/s]
Yt_max       = (Mf_max/wheelradius + Mr_max/wheelradius)*track;                    % maximum Yaw moment
PwrMax       = 80000;
PwrMin       = -40000;
maxSpeed     = 40;                        %m/sftire


%% Tire and suspension parameters
E = 0.23;
D = 1;
B = 0.3;
C = 1;


Sus_t = 10;                          % suspension time constant for 1st order system
tire_fxFactor = 1.5 ;                 % max Fx = Fz * tire_fxFactor
tire_fyFactor = 1.3 ;                 % max Fy = Fz * tire_fyFactor
%ftire = @(alph, Fz, p)(alph/pi*180)* Fz * tire_stifness ; %
%ftire = @(alph,Fz, p)  Fz* D*sin(C*atan(B*(alph/pi*180)  - E*atan(B*(alph/pi*180))));
ftire = @(alph, Fz)(alph./pi.*180)./15.* Fz .* tire_fyFactor ; %

%% Aerodynamics parameters
CL  = -4.15;
CD  = 1.55;
A   = 1;
COP = 0.5;    % Center of pressure on rear ratio
wingLength_f = 0.9;

%% environment parameters
g = 9.81;
airDensity = 1.225;


    Ft = u;

% Extract the controls from F
delta_f  = Ft(1);
delta_r  = Ft(2);
Fx_fl     = Ft(3);
Fx_fr     = Ft(4);
Fx_rl     = Ft(5);
Fx_rr     = Ft(6);


%% Extract the states from z
v_x  = z(1);
v_y  = z(2);
psi  = z(3);
dpsi = z(4);
X    = z(5);
Y    = z(6);
Fz   = z(7);

%% Compute the slip angles
%% Compute the slip angles
%% initialize matrices, origin of car is in COG
v = [v_x v_y 0];
dpsiv = [ 0 0 dpsi];
pos_fr = [  l_f  -track/2 0];
pos_fl = [  l_f   track/2 0];
pos_rr = [ -l_r -track/2 0];
pos_rl = [ -l_r  track/2 0];

%% Calculate vectors at uprights
velocityUpright_fl = v + cross(dpsiv,pos_fl);
velocityUpright_fr = v + cross(dpsiv,pos_fr);
velocityUpright_rl = v + cross(dpsiv,pos_rl);
velocityUpright_rr = v + cross(dpsiv,pos_rr);

%% Define Rotation matrices
rotate_f = [
    cos(delta_f) -sin(delta_f) 0
    sin(delta_f) cos(delta_f)  0
    0            0             0
    ];
rotate_r = [
    cos(delta_r) -sin(delta_r) 0
    sin(delta_r) cos(delta_r)  0
    0            0             0
    ];

%% Calculate wheel velocity in wheel frames
velocityWheel_fl = velocityUpright_fl * rotate_f;
velocityWheel_fr = velocityUpright_fr * rotate_f;
velocityWheel_rl = velocityUpright_rl * rotate_r;
velocityWheel_rr = velocityUpright_rr * rotate_r;


%% Calculate alphas
alpha_fl = -atan2(velocityWheel_fl(2),velocityWheel_fl(1));
alpha_fr = -atan2(velocityWheel_fr(2),velocityWheel_fr(1));
alpha_rl = -atan2(velocityWheel_rl(2),velocityWheel_rl(1));
alpha_rr = -atan2(velocityWheel_rr(2),velocityWheel_rr(1));


%% Compute the forces acting on the wheels
Fz_aero = 0.5*airDensity*CL*A*v_x.^2;
Fz_f = m/2*(1-COGr) * g - Fz/2 - Fz_aero/2 * (1-COP);
Fz_r = m/2*(COGr)   * g + Fz/2 - Fz_aero/2 * COP;

Fy_fl = ftire(alpha_fl,Fz_f);
Fy_fr = ftire(alpha_fr,Fz_f);
Fy_rl = ftire(alpha_rl,Fz_r);
Fy_rr = ftire(alpha_rr,Fz_r);

%% Projection of forces from steered wheels to uprights
projection_f = [
    cos(delta_f)      sin(delta_f)
    -sin(delta_f)     cos(delta_f)   
    ];
projection_r = [
    cos(delta_r)      sin(delta_r)
    -sin(delta_r)     cos(delta_r)   
    ];
%% Forces acting on uprights
F_fl = [Fx_fl Fy_fl] * projection_f;
F_fr = [Fx_fr Fy_fr] * projection_f;
F_rl = [Fx_rl Fy_rl] * projection_r;
F_rr = [Fx_rr Fy_rr] * projection_r;

F_drag = 0.5*airDensity*CD*A*v_x^2;
% Compute quantities need for the change of the position in the inertial frame
v = sqrt(v_x^2 + v_y^2);
beta = atan2(v_y, v_x);

M = (F_fr(1) + F_rr(1) - F_fl(1) - F_rl(1))*track/2 +... % Forward forces create Moment
    (F_fr(2) + F_fl(2)) * l_f...                         % Lateral forces from front tires
   -(F_rr(2) + F_rl(2)) * l_r;                          % Lateral forces from rear tires

Fx = F_fr(1) + F_rr(1) + F_fl(1) + F_rl(1)- F_drag;         % Longitudinal force from wheels and drag
Fy = F_fr(2) + F_rr(2) + F_fl(2) + F_rl(2);                  % Lateral force

aytest = Fy/m;
aytest2 = dpsi*v_x;
%dvx = 1/m  * (F_rx*cos(delta_r) - F_ry*sin(delta_r) + F_fx*cos(delta_f) - F_fy*sin(delta_f) - 0.5*airDensity*CD*A*v_x^2) + dpsi*v_y;
dz = [... 
Fx/m  + dpsi*v_y                                                                                                                      % v_x/dt
Fy/m  - dpsi*v_x                      % v_y/dt  
dpsi;                                                                                                                         % psi/dt
M/Izz   % dpsi
v*cos(psi + beta);                                                                                                            % X/dt
v*sin(psi + beta);                                                                                                            % Y/dt
((Fx/m + dpsi*v_y) *COGz/wheelbase*m-Fz)/Sus_t;                                                                              %Fz/dt  
];
end
